simulink model "pipelined_and_spatial_parallelism"  (R2015b)
settings: Solver=FixedStepDiscrete  SolverMode=SingleTasking  StartTime=0.0  StopTime=5e-4  RelTol=1e-3
undefined symbols (not defined in the file): a, b
libraries: shlslibv1 x5277
(part 23 of 23)

== system pipelined_and_spatial_parallelism/Simon_encrypt 3/Round_function8 ==
  " x_ii1" : Inport  OutMin=[0]  OutMax=[0]
  x_ii : Inport  Port=2  OutMin=[0]  OutMax=[0]
  k_i : Inport  Port=3  OutMin=[0]  OutMax=[0]
  Binary Logic : shlslibv1/Math Functions/Binary Logic  syn_binlog_exp=a&b  synBlockType=primitive  synLatency=0  synBlockId=13
  Binary Logic1 : shlslibv1/Math Functions/Binary Logic  syn_binlog_exp=a^b  synBlockType=primitive  synLatency=0  synBlockId=13
  Binary Logic2 : shlslibv1/Math Functions/Binary Logic  syn_binlog_exp=a^b  synBlockType=primitive  synLatency=0  synBlockId=13
  Binary Logic3 : shlslibv1/Math Functions/Binary Logic  syn_binlog_exp=a|b  synBlockType=primitive  synLatency=0  synBlockId=13
  Binary Logic4 : shlslibv1/Math Functions/Binary Logic  syn_binlog_exp=a^b  synBlockType=primitive  synLatency=0  synBlockId=13
  Binary Logic5 : shlslibv1/Math Functions/Binary Logic  syn_binlog_exp=a|b  synBlockType=primitive  synLatency=0  synBlockId=13
  Binary Logic6 : shlslibv1/Math Functions/Binary Logic  syn_binlog_exp=a|b  synBlockType=primitive  synLatency=0  synBlockId=13
  Constant : shlslibv1/Sources/Constant  syn_cst_val=1  syn_cst_format=Specify  syn_cst_wl=4  syn_cst_fl=0  syn_cst_dt=unsigned  syn_cst_rnd=on  syn_cst_st=-1  synBlockType=primitive  synLatency=0  synBlockId=15
  Constant1 : shlslibv1/Sources/Constant  syn_cst_val=8  syn_cst_format=Specify  syn_cst_wl=4  syn_cst_fl=0  syn_cst_dt=unsigned  syn_cst_rnd=on  syn_cst_st=-1  synBlockType=primitive  synLatency=0  synBlockId=15
  Constant2 : shlslibv1/Sources/Constant  syn_cst_val=2  syn_cst_format=Specify  syn_cst_wl=4  syn_cst_fl=0  syn_cst_dt=unsigned  syn_cst_rnd=on  syn_cst_st=-1  synBlockType=primitive  synLatency=0  synBlockId=15
  Constant3 : shlslibv1/Sources/Constant  syn_cst_val=15  syn_cst_format=Specify  syn_cst_wl=4  syn_cst_fl=0  syn_cst_dt=unsigned  syn_cst_rnd=on  syn_cst_st=-1  synBlockType=primitive  synLatency=0  synBlockId=15
  Constant4 : shlslibv1/Sources/Constant  syn_cst_val=8  syn_cst_format=Specify  syn_cst_wl=4  syn_cst_fl=0  syn_cst_dt=unsigned  syn_cst_rnd=on  syn_cst_st=-1  synBlockType=primitive  synLatency=0  synBlockId=15
  Constant5 : shlslibv1/Sources/Constant  syn_cst_val=14  syn_cst_format=Specify  syn_cst_wl=4  syn_cst_fl=0  syn_cst_dt=unsigned  syn_cst_rnd=on  syn_cst_st=-1  synBlockType=primitive  synLatency=0  synBlockId=15
  Shifter : shlslibv1/Math Functions/Shifter  syn_shifter_opr=<<  syn_out_f=Automatic  syn_out_wl=16  syn_out_fl=8  syn_out_dt=signed  synBlockType=primitive  synLatency=0  synBlockId=12
  Shifter1 : shlslibv1/Math Functions/Shifter  syn_shifter_opr=>>  syn_out_f=Automatic  syn_out_wl=16  syn_out_fl=8  syn_out_dt=signed  synBlockType=primitive  synLatency=0  synBlockId=12
  Shifter2 : shlslibv1/Math Functions/Shifter  syn_shifter_opr=<<  syn_out_f=Automatic  syn_out_wl=16  syn_out_fl=8  syn_out_dt=signed  synBlockType=primitive  synLatency=0  synBlockId=12
  Shifter3 : shlslibv1/Math Functions/Shifter  syn_shifter_opr=>>  syn_out_f=Automatic  syn_out_wl=16  syn_out_fl=8  syn_out_dt=signed  synBlockType=primitive  synLatency=0  synBlockId=12
  Shifter4 : shlslibv1/Math Functions/Shifter  syn_shifter_opr=<<  syn_out_f=Automatic  syn_out_wl=16  syn_out_fl=8  syn_out_dt=signed  synBlockType=primitive  synLatency=0  synBlockId=12
  Shifter5 : shlslibv1/Math Functions/Shifter  syn_shifter_opr=>>  syn_out_f=Automatic  syn_out_wl=16  syn_out_fl=8  syn_out_dt=signed  synBlockType=primitive  synLatency=0  synBlockId=12
  Xiii1 : Outport
  xiii2 : Outport  Port=2
  wires:
  Binary Logic/1 -> Binary Logic2/2
  Binary Logic2/1 -> Binary Logic4/1
  Binary Logic4/1 -> Binary Logic1/1
  Constant/1 -> Shifter/2
  Constant1/1 -> Shifter2/2
  Binary Logic1/1 -> xiii2/1
  x_ii/1 -> Binary Logic2/1
  " x_ii1"/1 -> Shifter/1, Shifter1/1, Shifter2/1, Shifter3/1, Shifter4/1, Xiii1/1, Shifter5/1
  k_i/1 -> Binary Logic1/2
  Constant3/1 -> Shifter1/2
  Shifter/1 -> Binary Logic3/1
  Shifter1/1 -> Binary Logic3/2
  Binary Logic3/1 -> Binary Logic/1
  Constant4/1 -> Shifter3/2
  Shifter2/1 -> Binary Logic5/1
  Shifter3/1 -> Binary Logic5/2
  Binary Logic5/1 -> Binary Logic/2
  Constant2/1 -> Shifter4/2
  Shifter4/1 -> Binary Logic6/1
  Constant5/1 -> Shifter5/2
  Shifter5/1 -> Binary Logic6/2
  Binary Logic6/1 -> Binary Logic4/2

== system pipelined_and_spatial_parallelism/Simon_encrypt 3/Round_function9 ==
  " x_ii1" : Inport  OutMin=[0]  OutMax=[0]
  x_ii : Inport  Port=2  OutMin=[0]  OutMax=[0]
  k_i : Inport  Port=3  OutMin=[0]  OutMax=[0]
  Binary Logic : shlslibv1/Math Functions/Binary Logic  syn_binlog_exp=a&b  synBlockType=primitive  synLatency=0  synBlockId=13
  Binary Logic1 : shlslibv1/Math Functions/Binary Logic  syn_binlog_exp=a^b  synBlockType=primitive  synLatency=0  synBlockId=13
  Binary Logic2 : shlslibv1/Math Functions/Binary Logic  syn_binlog_exp=a^b  synBlockType=primitive  synLatency=0  synBlockId=13
  Binary Logic3 : shlslibv1/Math Functions/Binary Logic  syn_binlog_exp=a|b  synBlockType=primitive  synLatency=0  synBlockId=13
  Binary Logic4 : shlslibv1/Math Functions/Binary Logic  syn_binlog_exp=a^b  synBlockType=primitive  synLatency=0  synBlockId=13
  Binary Logic5 : shlslibv1/Math Functions/Binary Logic  syn_binlog_exp=a|b  synBlockType=primitive  synLatency=0  synBlockId=13
  Binary Logic6 : shlslibv1/Math Functions/Binary Logic  syn_binlog_exp=a|b  synBlockType=primitive  synLatency=0  synBlockId=13
  Constant : shlslibv1/Sources/Constant  syn_cst_val=1  syn_cst_format=Specify  syn_cst_wl=4  syn_cst_fl=0  syn_cst_dt=unsigned  syn_cst_rnd=on  syn_cst_st=-1  synBlockType=primitive  synLatency=0  synBlockId=15
  Constant1 : shlslibv1/Sources/Constant  syn_cst_val=8  syn_cst_format=Specify  syn_cst_wl=4  syn_cst_fl=0  syn_cst_dt=unsigned  syn_cst_rnd=on  syn_cst_st=-1  synBlockType=primitive  synLatency=0  synBlockId=15
  Constant2 : shlslibv1/Sources/Constant  syn_cst_val=2  syn_cst_format=Specify  syn_cst_wl=4  syn_cst_fl=0  syn_cst_dt=unsigned  syn_cst_rnd=on  syn_cst_st=-1  synBlockType=primitive  synLatency=0  synBlockId=15
  Constant3 : shlslibv1/Sources/Constant  syn_cst_val=15  syn_cst_format=Specify  syn_cst_wl=4  syn_cst_fl=0  syn_cst_dt=unsigned  syn_cst_rnd=on  syn_cst_st=-1  synBlockType=primitive  synLatency=0  synBlockId=15
  Constant4 : shlslibv1/Sources/Constant  syn_cst_val=8  syn_cst_format=Specify  syn_cst_wl=4  syn_cst_fl=0  syn_cst_dt=unsigned  syn_cst_rnd=on  syn_cst_st=-1  synBlockType=primitive  synLatency=0  synBlockId=15
  Constant5 : shlslibv1/Sources/Constant  syn_cst_val=14  syn_cst_format=Specify  syn_cst_wl=4  syn_cst_fl=0  syn_cst_dt=unsigned  syn_cst_rnd=on  syn_cst_st=-1  synBlockType=primitive  synLatency=0  synBlockId=15
  Shifter : shlslibv1/Math Functions/Shifter  syn_shifter_opr=<<  syn_out_f=Automatic  syn_out_wl=16  syn_out_fl=8  syn_out_dt=signed  synBlockType=primitive  synLatency=0  synBlockId=12
  Shifter1 : shlslibv1/Math Functions/Shifter  syn_shifter_opr=>>  syn_out_f=Automatic  syn_out_wl=16  syn_out_fl=8  syn_out_dt=signed  synBlockType=primitive  synLatency=0  synBlockId=12
  Shifter2 : shlslibv1/Math Functions/Shifter  syn_shifter_opr=<<  syn_out_f=Automatic  syn_out_wl=16  syn_out_fl=8  syn_out_dt=signed  synBlockType=primitive  synLatency=0  synBlockId=12
  Shifter3 : shlslibv1/Math Functions/Shifter  syn_shifter_opr=>>  syn_out_f=Automatic  syn_out_wl=16  syn_out_fl=8  syn_out_dt=signed  synBlockType=primitive  synLatency=0  synBlockId=12
  Shifter4 : shlslibv1/Math Functions/Shifter  syn_shifter_opr=<<  syn_out_f=Automatic  syn_out_wl=16  syn_out_fl=8  syn_out_dt=signed  synBlockType=primitive  synLatency=0  synBlockId=12
  Shifter5 : shlslibv1/Math Functions/Shifter  syn_shifter_opr=>>  syn_out_f=Automatic  syn_out_wl=16  syn_out_fl=8  syn_out_dt=signed  synBlockType=primitive  synLatency=0  synBlockId=12
  Xiii1 : Outport
  xiii2 : Outport  Port=2
  wires:
  Binary Logic/1 -> Binary Logic2/2
  Binary Logic2/1 -> Binary Logic4/1
  Binary Logic4/1 -> Binary Logic1/1
  Constant/1 -> Shifter/2
  Constant1/1 -> Shifter2/2
  Binary Logic1/1 -> xiii2/1
  x_ii/1 -> Binary Logic2/1
  " x_ii1"/1 -> Shifter/1, Shifter1/1, Shifter2/1, Shifter3/1, Shifter4/1, Xiii1/1, Shifter5/1
  k_i/1 -> Binary Logic1/2
  Constant3/1 -> Shifter1/2
  Shifter/1 -> Binary Logic3/1
  Shifter1/1 -> Binary Logic3/2
  Binary Logic3/1 -> Binary Logic/1
  Constant4/1 -> Shifter3/2
  Shifter2/1 -> Binary Logic5/1
  Shifter3/1 -> Binary Logic5/2
  Binary Logic5/1 -> Binary Logic/2
  Constant2/1 -> Shifter4/2
  Shifter4/1 -> Binary Logic6/1
  Constant5/1 -> Shifter5/2
  Shifter5/1 -> Binary Logic6/2
  Binary Logic6/1 -> Binary Logic4/2
